simulink model "TV_2020_v1_TCELDAS_YAW_1_FUNregenerativa_ETAS"  (R2017b)
settings: Solver=ode3  StartTime=0  StopTime=10  FixedStep=0.05  RelTol=1e-3  EnableMultiTasking=on
(part 5 of 5)

== matlab function TV_2020_v1_TCELDAS_YAW_1_FUNregenerativa_ETAS/Vehicle Dynamics Control 2018/VDC 2018 Complete/Optimization SKF & CKF/Subsystem /MATLAB Function1 ==
  data: cte input; v input; value output
function value = switch_fcn(cte,v)
if v > cte;
    value = cte;
elseif v < -cte;
    value = -cte;
else
    value = v;
end

== matlab function TV_2020_v1_TCELDAS_YAW_1_FUNregenerativa_ETAS/Vehicle Dynamics Control 2018/VDC 2018 Complete/Optimization SKF & CKF/Subsystem /SKF/No spin/MATLAB Function ==
  data: SKF_prev input; SKF_Initial input; SKF_act0 output
function SKF_act0 = fcn(SKF_prev, SKF_Initial)

if SKF_prev < SKF_Initial
SKF_act0 = SKF_prev;

else
SKF_act0 = SKF_Initial;

end

== matlab function TV_2020_v1_TCELDAS_YAW_1_FUNregenerativa_ETAS/Vehicle Dynamics Control 2018/VDC 2018 Complete/Optimization SKF & CKF/Subsystem /SKF/Spin/MATLAB Function ==
  data: SKF_Initial input; SKF_act1 output; SKF_prev input
function SKF_act1 = fcn(SKF_Initial, SKF_prev)

if SKF_prev < SKF_Initial
SKF_act1 = SKF_prev;

else
SKF_act1 = SKF_Initial;

end

== matlab function TV_2020_v1_TCELDAS_YAW_1_FUNregenerativa_ETAS/Vehicle Dynamics Control 2018/VDC 2018 without Longitudinal/Optimization SKF & CKF/MATLAB Function ==
  data: RPM_INV1 input; RPM output; RPM_INV2 input
function RPM = fcn(RPM_INV1, RPM_INV2)

if RPM_INV1 > RPM_INV2
RPM = RPM_INV1;

else
RPM = RPM_INV2;

end

== matlab function TV_2020_v1_TCELDAS_YAW_1_FUNregenerativa_ETAS/Vehicle Dynamics Control 2018/VDC 2018 without Longitudinal/Optimization SKF & CKF/Subsystem /CKF/No spin/MATLAB Function ==
  data: CKF_prev input; CKF_act0 output; CKF_Initial input
function CKF_act0 = fcn(CKF_prev, CKF_Initial)

if CKF_prev < CKF_Initial
CKF_act0 = CKF_prev;

else
CKF_act0 = CKF_Initial;

end

== matlab function TV_2020_v1_TCELDAS_YAW_1_FUNregenerativa_ETAS/Vehicle Dynamics Control 2018/VDC 2018 without Longitudinal/Optimization SKF & CKF/Subsystem /CKF/Spin /MATLAB Function ==
  data: CKF_Initial input; CKF_act1 output; CKF_prev input
function CKF_act1 = fcn(CKF_Initial, CKF_prev)

if CKF_prev < CKF_Initial
CKF_act1 = CKF_prev;

else
CKF_act1 = CKF_Initial;

end

== matlab function TV_2020_v1_TCELDAS_YAW_1_FUNregenerativa_ETAS/Vehicle Dynamics Control 2018/VDC 2018 Complete/Lateral Dynamics/Yaw_Rate_Reference/Bicycle Model ==
  data: delta input; r output; vx input; beta output; alpha_f output; alpha_r output; course output; radius output; yf output; yr output; m input; xCG input; L input; cf input; cr input
function [r,beta,alpha_f,alpha_r,course,radius,yf,yr]...
    = fcn(delta,vx,m,xCG,L,cf,cr)
% OTHER CONSTANTS
lf = xCG;
lr = L - xCG;

% INPUTS TO STANDARD UNITS
delta = delta*2*pi/360;           % º to rad

% CALCULATIONS    (Outputs are in SI units)
A = [cf, cr, -m*vx
    lf*cf, -lr*cr, 0
    -1, 1, L/vx];
B = [0; 0; delta];
X = A\B; 

alpha_f = X(1,1);                 
alpha_r = X(2,1);                  
r = X(3,1);                     
course = alpha_f + delta;

vx_f = vx;
vx_r = vx;
vy_r = vx_r*tan(alpha_r);
vy_f = vx_f*tan(alpha_f + delta); 
vy = vy_r + r*lr;

beta = atan(vy/vx);
beta(isnan(beta)) = 0;
v = vx/cos(beta);

radius = vx/r; 

yf = cf*alpha_f;
yr = cr*alpha_r;
fy = yf + yr;

alphadiff_ay = (-alpha_f + alpha_r)/((vx)^2/radius)*360/(2*pi);    % Slip Angle diff respect to Lateral Acceleration [º/N]

== matlab function TV_2020_v1_TCELDAS_YAW_1_FUNregenerativa_ETAS/Vehicle Dynamics Control 2018/VDC 2018 Complete/Lateral Dynamics/Force Difference with Max. Tire Forces ==
  data: fx_diff input; rr_fx output; rr_fx_max input; rl_fx_max input; rl_fx output
function [rr_fx, rl_fx]= fcn(fx_diff, rr_fx_max, rl_fx_max)

if fx_diff > 0      % Momento hacia derechas
    rl_fx = rl_fx_max;
    rr_fx = rl_fx - fx_diff;
    if rr_fx > rr_fx_max
        rr_fx = rr_fx_max;  % Control de tracción
        rl_fx = rr_fx + fx_diff;  % OJO: No estamos trabajando al límite de los neumáticos
    end
    
elseif fx_diff < 0  % Momento hacia izquierdas
    rr_fx = rr_fx_max;
    rl_fx = rr_fx - abs(fx_diff);
    if rl_fx > rl_fx_max
        rl_fx = rl_fx_max;  % Control de tracción
        rr_fx = rl_fx - abs(fx_diff);  % OJO: No estamos trabajando al límite de los neumáticos
    end
    
else                % Momento nulo - Escoger par mínimo RL
    if rr_fx_max > rl_fx_max
        rl_fx = rl_fx_max;
        rr_fx = rl_fx;
    elseif rr_fx_max < rl_fx_max
        rr_fx = rr_fx_max;
        rl_fx = rr_fx;
    else
        rr_fx = rr_fx_max;
        rl_fx = rr_fx;
    end
end

== matlab function TV_2020_v1_TCELDAS_YAW_1_FUNregenerativa_ETAS/Vehicle Dynamics Control 2018/VDC 2018 Complete/Constraints/Acelerating and braking without Regenerative/MATLAB Function ==
  data: diff_wc input; diff_lim output; diff_max input
function diff_lim = fcn(diff_wc,diff_max)

if diff_wc < -diff_max
    diff_lim = -diff_max;
elseif diff_wc > diff_max
    diff_lim = diff_max;
else
    diff_lim = diff_wc;
end
